simulink model "ProjectOfPreCrashSafetySystem"  (R2016b)
settings: Solver=VariableStepAuto  StartTime=0.0  StopTime=10.0  RelTol=1e-3
settings Model: Creator=Takiya  LastModifiedBy=Takiya

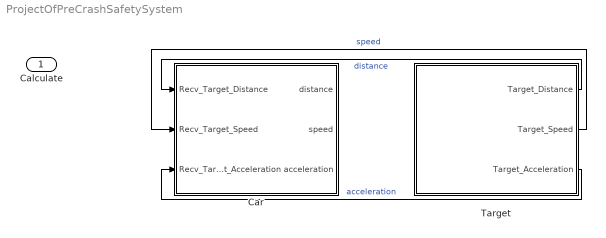
== system ProjectOfPreCrashSafetySystem ==
  Calculate : Inport
      settings: AttributesFormatString=ECU_Calculating
  Car : Subsystem
  Target : Subsystem
      settings: AttributesFormatString=TargetCar
  wires:
  Target/3(Target_Acceleration) -> Car/3(Recv_Target_Acceleration)  "acceleration"
  Target/1(Target_Distance) -> Car/1(Recv_Target_Distance)  "distance"
  Target/2(Target_Speed) -> Car/2(Recv_Target_Speed)  "speed"

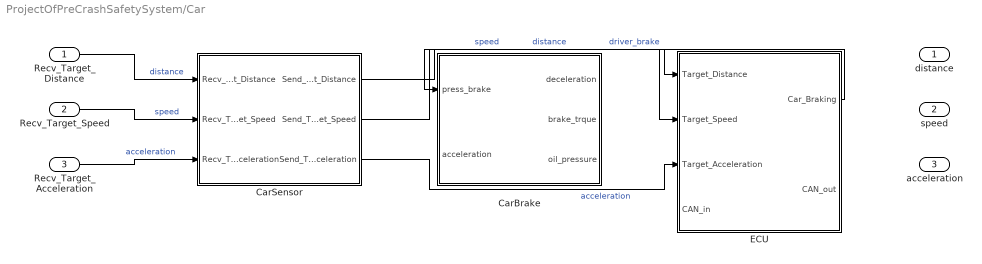
== system ProjectOfPreCrashSafetySystem/Car ==
  Recv_Target_Distance : Inport
      settings: AttributesFormatString=distance
  Recv_Target_Speed : Inport  Port=2
      settings: AttributesFormatString=speed
  Recv_Target_Acceleration : Inport  Port=3
      settings: AttributesFormatString=acceleration
  CarBrake : Subsystem
      settings: AttributesFormatString=Brake
  CarSensor : Subsystem
      settings: AttributesFormatString=Sensor
  ECU : Subsystem
  distance : Outport
  speed : Outport  Port=2
  acceleration : Outport  Port=3
  wires:
  CarSensor/3(Send_Target_Acceleration) -> ECU/3(Target_Acceleration)  "acceleration"
  CarSensor/1(Send_Target_Distance) -> ECU/1(Target_Distance)  "distance"
  CarSensor/2(Send_Target_Speed) -> ECU/2(Target_Speed)  "speed"
  ECU/1(Car_Braking) -> CarBrake/1(press_brake)  "driver_brake"
  Recv_Target_Distance/1 -> CarSensor/1(Recv_Target_Distance)  "distance"
  Recv_Target_Speed/1 -> CarSensor/2(Recv_Target_Speed)  "speed"
  Recv_Target_Acceleration/1 -> CarSensor/3(Recv_Target_Acceleration)  "acceleration"

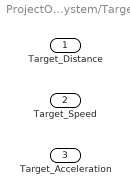
== system ProjectOfPreCrashSafetySystem/Target ==
  Target_Distance : Outport
      settings: AttributesFormatString=distance
  Target_Speed : Outport  Port=2
      settings: AttributesFormatString=speed
  Target_Acceleration : Outport  Port=3
      settings: AttributesFormatString=acceleration

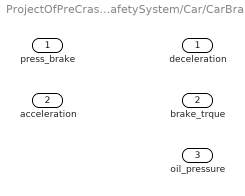
== system ProjectOfPreCrashSafetySystem/Car/CarBrake ==
  press_brake : Inport
      settings: AttributesFormatString=driver_brake
  acceleration : Inport  Port=2
  deceleration : Outport
      settings: AttributesFormatString=acceleration
  brake_trque : Outport  Port=2
      settings: AttributesFormatString=trque
  oil_pressure : Outport  Port=3
      settings: AttributesFormatString=press

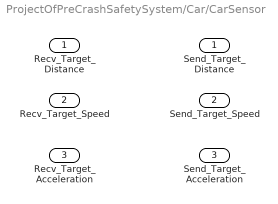
== system ProjectOfPreCrashSafetySystem/Car/CarSensor ==
  Recv_Target_Distance : Inport
      settings: AttributesFormatString=distance
  Recv_Target_Speed : Inport  Port=2
      settings: AttributesFormatString=speed
  Recv_Target_Acceleration : Inport  Port=3
      settings: AttributesFormatString=acceleration
  Send_Target_Distance : Outport
      settings: AttributesFormatString=distance
  Send_Target_Speed : Outport  Port=2
      settings: AttributesFormatString=speed
  Send_Target_Acceleration : Outport  Port=3
      settings: AttributesFormatString=acceleration

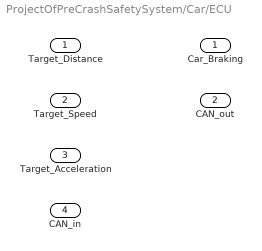
== system ProjectOfPreCrashSafetySystem/Car/ECU ==
  Target_Distance : Inport
      settings: AttributesFormatString=distance
  Target_Speed : Inport  Port=2
      settings: AttributesFormatString=speed
  Target_Acceleration : Inport  Port=3
      settings: AttributesFormatString=acceleration
  CAN_in : Inport  Port=4
      settings: AttributesFormatString=CAN_DATA
  Car_Braking : Outport
      settings: AttributesFormatString=driver_brake
  CAN_out : Outport  Port=2
      settings: AttributesFormatString=CAN_DATA
